simulink model "option3"  (R2023b)
settings: Solver=VariableStepAuto  StartTime=0.0  StopTime=10.0  RelTol=1e-3
values from neighbouring files (symbols this model uses):
  b1 = 1    [combined_options_code.m]    (also in option1_code.m; option2_code.m; option3_code.m)
  b2 = 1    [combined_options_code.m]    (also in option1_code.m; option2_code.m; option3_code.m)
  J1 = 100    [combined_options_code.m]    (also in option1_code.m; option2_code.m; option3_code.m)
  J2 = 1    [combined_options_code.m]    (also in option1_code.m; option2_code.m; option3_code.m)
  torque_iteration = A_constant_torque_S1(x)    [combined_options_code.m]    (also in option1_code.m; option2_code.m; option3_code.m)
  torque_iteration2 = A_constant_torque_S2(x)    [combined_options_code.m]    (also in option1_code.m; option2_code.m; option3_code.m)
settings Model: Creator=Conor  LastModifiedBy=Conor

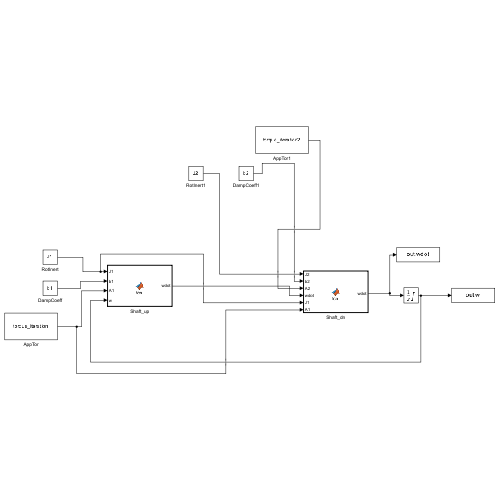
[thumbnail: Simulink's stored preview of the top-level diagram]
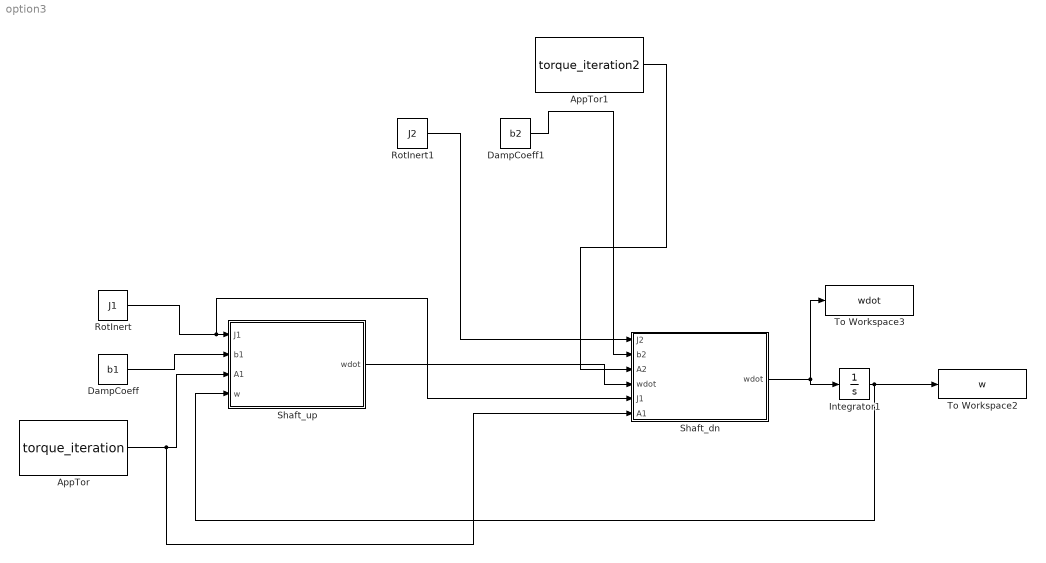
== system option3 ==
  AppTor : Constant  Value=torque_iteration
  AppTor1 : Constant  Value=torque_iteration2
  DampCoeff : Constant  Value=b1
  DampCoeff1 : Constant  Value=b2
  Integrator1 : Integrator  LimitOutput=on  UpperSaturationLimit=10
  RotInert : Constant  Value=J1  SampleTime=-1
  RotInert1 : Constant  Value=J2  SampleTime=-1
  Shaft_dn : MATLAB Function  TreatAsAtomicUnit=on
  Shaft_up : MATLAB Function  TreatAsAtomicUnit=on
  To Workspace2 : ToWorkspace  VariableName=w  SaveFormat=Timeseries  SampleTime=-1
  To Workspace3 : ToWorkspace  VariableName=wdot  SaveFormat=Timeseries  SampleTime=-1
  wires:
  RotInert/1 -> Shaft_dn/5(J1), Shaft_up/1(J1)
  DampCoeff/1 -> Shaft_up/2(b1)
  AppTor/1 -> Shaft_up/3(A1), Shaft_dn/6(A1)
  Shaft_up/1(wdot) -> Shaft_dn/4("wdot ")
  AppTor1/1 -> Shaft_dn/3(A2)
  Shaft_dn/1(wdot) -> To Workspace3/1, Integrator1/1
  Integrator1/1 -> Shaft_up/4(w), To Workspace2/1
  RotInert1/1 -> Shaft_dn/1(J2)
  DampCoeff1/1 -> Shaft_dn/2(b2)

== matlab function option3/Shaft_dn ==
  data: J2 input; wdot output; b2 input; A2 input; wdot input; J1 input; A1 input
function wdot = fcn(J2, b2, A2, wdot, J1, A1)

wdot = (A1 + J1*wdot - A2)/(J1+J2);

== matlab function option3/Shaft_up ==
  data: J1 input; wdot output; b1 input; A1 input; w input
function wdot = fcn(J1, b1, A1, w)

wdot = (1 / J1) * (A1 - b1*w);
